simulink model "Dyn_6DoF_v2_0_R2015B"  (R2015b)
settings: Solver=ode4  SolverMode=SingleTasking  StartTime=0.0  StopTime=simInit.TSIM  FixedStep=simInit.dt  MaxStep=simInit.dt  RelTol=1e-3
InitFcn:
  | close all
undefined symbols (not defined in the file): act, base_windspeed, constr, DE2019, DiscIntNeverNeededParam, ENVMT, Lbooth, loiterStates, omega_rate_max, params, simInit, T, winchParameter
libraries: simulink x41, simulink_extras x4, dspsigops x1
(part 6 of 6)

== matlab function Dyn_6DoF_v2_0_R2015B/AirborneSystem/FlightControlSystem/PathFollowingController_SS_3/FlightOnFlatEarth (Retraction&Loitering)/CalculateAttitudeCmds/FlightPathLoopRetraction_Aerodynamic/TrafoPathKin2PathAero ==
  data: Va input; beta input; Vg input; v_w_O input; chi_k input; gamma_k input; chi_a output; gamma_a output
% Copyright 2021 Delft University of Technology
%
% Licensed under the Apache License, Version 2.0 (the "License");
% you may not use this file except in compliance with the License.
% You may obtain a copy of the License at
%
%      http://www.apache.org/licenses/LICENSE-2.0
%
% Unless required by applicable law or agreed to in writing, software
% distributed under the License is distributed on an "AS IS" BASIS,
% WITHOUT WARRANTIES OR CONDITIONS OF ANY KIND, either express or implied.
% See the License for the specific language governing permissions and
% limitations under the License.

function [chi_a, gamma_a] = PathKin2PathAero(Va, beta, Vg, v_w_O, chi_k, gamma_k)
%PathKin2PathAero - transform kinetic path angles into aerodynamic path
%                   angles
%
% Inputs:
%    Va         - Aircraft velocity component on body x axis
%    beta       - Aircraft side slip angle
%    Vg         - Kinetic velocity magnitude
%    v_w_O      - Wind velocity at aircraft in inertial reference frame
%    chi_k      - Kinetic course heading
%    gamma_k    - Kinetic path angle
%
% Outputs:
%    chi_a      - Aerodynamic course heading
%    gamma_a 	- Aerodynamic path angle
%
% Example: [chi_a, gamma_a] = fcn(Va, beta, Vg, v_w_O, chi_k, gamma_k)
%
% Other m-files required: none
% Subfunctions: none
% MAT-files required: none
%
% Author: Sebastian Rapp, Phd.
% Delft University of Technology
% email address: s.rapp@tudelft.nl  

%------------- BEGIN CODE --------------
gamma_a = asin( max( min( (Vg*sin(gamma_k)+v_w_O(3))/(Va+1e-9),1), -1) );
chi_a = beta + chi_k - asin( max( min( 1/(Va*cos(gamma_a)) * (v_w_O(1)*(-sin(chi_k))+v_w_O(2)*cos(chi_k)),1), -1) );
%------------- END CODE --------------
end

== matlab function Dyn_6DoF_v2_0_R2015B/AirborneSystem/ForcesAndTorques/aerodynamic forces FSI/Wing Aero/If Action Subsystem1/FSI/Simple_wing_aero ==
  data: input input double; out output double size=[6,1]; DE2019 parameter; ENVMT parameter
% Copyright 2021 Delft University of Technology
%
% Licensed under the Apache License, Version 2.0 (the "License");
% you may not use this file except in compliance with the License.
% You may obtain a copy of the License at
%
%      http://www.apache.org/licenses/LICENSE-2.0
%
% Unless required by applicable law or agreed to in writing, software
% distributed under the License is distributed on an "AS IS" BASIS,
% WITHOUT WARRANTIES OR CONDITIONS OF ANY KIND, either express or implied.
% See the License for the specific language governing permissions and
% limitations under the License.

function out = simpleAero(input, DE2019, ENVMT)
%simpleAero - Main wing simple aero calculation
%
% Inputs:
%    input  - airspeed, AoA, CL, CD, CM and Croll
%    DE2019 - Aircraft parameters
%    ENVMT  - Environment characteristics
%
% Outputs:
%    out    - 3D forces and moments generated by the wing
%
%
% Author: Sebastian Rapp, Ph.D., Revised by: Dylan Eijkelhof, M.Sc.
% Delft University of Technology
% email address: d.eijkelhof@tudelft.nl
% December 2019; Last revision: 19-March-2021

%-------------	BEGIN CODE	--------------
    V = input(1);
    alpha = input(2);

    q = 0.5*ENVMT.rhos*V^2;

    F_L_main = -input(3)*q*DE2019.S_ref;
    F_D_main = input(4)*q*DE2019.S_ref;
    
    M_y_mw = input(5)*q*DE2019.S_wing*DE2019.c + ...
        (0.25*DE2019.c+DE2019.cog(1))*F_L_main;
    
    c_roll_mw = input(6);
    M_x_mw = (c_roll_mw) * q * DE2019.S_wing * DE2019.b;
    
    F_x_mw = -F_D_main*cos(alpha) - F_L_main*sin(alpha);
    F_z_mw = F_L_main*cos(alpha);


    out = [F_x_mw, 0, F_z_mw, M_x_mw, M_y_mw, 0]';
%-------------	END CODE	--------------
end

== stateflow chart Dyn_6DoF_v2_0_R2015B/AirborneSystem/FlightControlSystem/PathFollowingController_SS_3/FlightOnFlatEarth (Retraction&Loitering)/GuidanceFlatEarth/LoiteringGuidance/Loiter ==
  state initLoiter
    during: [e_track,course_des,valid_transition_region_flag]  = initLoiterGuidance(kp_course_init, p_x_W,p_y_W, pos_OLoiter_W, R_init_loiter, windDir, Vk, validTransReg_start, validTransReg_end);
  (default) -> (junction 217)
  (junction 217) -> initLoiter : [1]
  data: delta function_output; kp_ function_input; p_x_W_ function_input; p_y_W_ function_input; pos_OLoiter_W_ function_input; R_ function_input; windDirection_rad_ function_input; Vk_ function_input; course_des_ function_output; valid_transition_region_flag_ function_output; validTransReg_start_ function_input; validTransReg_end_ function_input; course_des output; p_y_W input; course_k input; p_x_W input; Vk input; kp_course_init parameter; validTransReg_start parameter; validTransReg_end parameter; pos_OLoiter_W parameter; R_init_loiter parameter; valid_transition_region_flag output; e_track output; reset_flag input; windDir input
  function [delta, course_des_,valid_transition_region_flag_]  = initLoiterGuidance(kp_, p_x_W_,p_y_W_, pos_OLoiter_W_, R_, windDirection_rad_, Vk_, validTransReg_start_, validTransReg_end_):
    | % Copyright 2020 Delft University of Technology
    | %
    | % Licensed under the Apache License, Version 2.0 (the "License");
    | % you may not use this file except in compliance with the License.
    | % You may obtain a copy of the License at
    | %
    | %      http://www.apache.org/licenses/LICENSE-2.0
    | %
    | % Unless required by applicable law or agreed to in writing, software
    | % distributed under the License is distributed on an "AS IS" BASIS,
    | % WITHOUT WARRANTIES OR CONDITIONS OF ANY KIND, either express or implied.
    | % See the License for the specific language governing permissions and
    | % limitations under the License. 
    | 
    | function [delta, course_des_,valid_transition_region_flag_]  = initLoiterGuidance(kp_, p_x_W_,p_y_W_, pos_OLoiter_W_, R_, windDirection_rad_, Vk_, validTransReg_start_, validTransReg_end_) 
    | 
    | %#codegen
    | 
    | %% LOITER GUIDANCE: compare with approach where height and ground track is controlled independently
    | p_W_ = [p_x_W_; p_y_W_; 0];
    | 
    | pos_OLoiter_W_(3) = 0;
    | r_circ_W =  pos_OLoiter_W_;
    | 
    | 
    | p_P =  ( p_W_ - r_circ_W );
    | V = [1, 0; 0, 1; 0, 0];
    | p_P = V*((V'*V)\eye(2))*V'*p_P;
    | p_P = p_P / norm(p_P) * R_;
    | 
    | s_star = atan2( p_P(2), p_P(1) );
    | t_P = [-sin(s_star); cos(s_star); 0]*R_;
    | t_W = t_P;% + r_circ_W;
    | t_O = transformFromWtoO(windDirection_rad_, t_W);
    | 
    | p_proj_W =  p_P + r_circ_W;
    | delta_W = p_W_ - p_proj_W;
    | delta = norm( delta_W );
    | 
    | 
    | epx = t_W/norm(t_W);
    | epy = delta_W/norm(delta_W);
    | epz = cross( epx, epy ); epz = epz/norm(epz);
    | 
    | chi_star = atan2(t_O(2), t_O(1));
    | deltaChi = sign(epz(3))*asin( max( min( delta*kp_/Vk_ ,1),-1) );  %atan2( delta, 0.1*R_ );
    | 
    | course_des_ = chi_star + deltaChi;
    | 
    | bearing_O = [cos(course_des_); sin(course_des_); 0];
    | bearing_W = transformFromOtoW(windDirection_rad_, bearing_O);
    | 
    | if s_star > validTransReg_start_ && s_star < validTransReg_end_
    |     valid_transition_region_flag_ = 1;
    | else
    |     valid_transition_region_flag_ = 0;
    | end

== matlab function Dyn_6DoF_v2_0_R2015B/AirborneSystem/6DoFDynamics/MATLAB Function3 ==
  data: v_w_O output; v_w_W input; ENVMT parameter
% Copyright 2021 Delft University of Technology
%
% Licensed under the Apache License, Version 2.0 (the "License");
% you may not use this file except in compliance with the License.
% You may obtain a copy of the License at
%
%      http://www.apache.org/licenses/LICENSE-2.0
%
% Unless required by applicable law or agreed to in writing, software
% distributed under the License is distributed on an "AS IS" BASIS,
% WITHOUT WARRANTIES OR CONDITIONS OF ANY KIND, either express or implied.
% See the License for the specific language governing permissions and
% limitations under the License.

function v_w_O = fcn(v_w_W, ENVMT)

v_w_O = transformFromWtoO(ENVMT.windDirection_rad, v_w_W );
end

== stateflow chart Dyn_6DoF_v2_0_R2015B/GroundSystem_SS_6/StateMachine/checkRetractionCondition ==
  state calcIncrement1
    during: l_tether_predict =l_tether+l_tether-l0;
  state init2
    entry: init_retraction_flag=1;
  state init
    entry: init_retraction_flag=0;
  state calcIncrement
    during: l_tether_predict =l_tether+l_tether-l0;
  state set0length
    entry: l0 = l_tether;
  calcIncrement1 -> (junction 38) : [path_parameter_s >= (3*pi/2-1*pi/180) && path_parameter_s <=3*pi/2+1*pi/180 ]
  init2 -> init : [fm==6]
  (junction 38) -> init2 [order 1] : [l_tether_predict>=l_tether_max*1.15]
  set0length -> calcIncrement1 [order 4] : [path_parameter_s >= (pi/2-1*pi/180) && path_parameter_s <= pi/2+1*pi/180]
  (default) -> init
  set0length -> init [order 2] : [fm==6]
  (junction 38) -> set0length [order 2]
  calcIncrement -> (junction 38) : [path_parameter_s >= (pi/2-1*pi/180) && path_parameter_s <= pi/2+1*pi/180]
  set0length -> init [order 3] : [fm==6]
  init -> set0length : [path_parameter_s >= (pi/2-1*pi/180) && path_parameter_s <= pi/2+1*pi/180 &&fm==5]
  set0length -> calcIncrement [order 1] : [path_parameter_s >= (3*pi/2-1*pi/180) && path_parameter_s <=3*pi/2+1*pi/180 ]
  data: l_tether input; path_parameter_s input; fm input; l0 local; init_retraction_flag output; l_tether_max input; dl local; l_tether_predict local

== matlab function Dyn_6DoF_v2_0_R2015B/AirborneSystem/FlightControlSystem/PathFollowingController_SS_3/FlightOnFlatEarth (Retraction&Loitering)/GuidanceFlatEarth/Retraction_Nav/MATLAB Function1 ==
  data: vel_k_O input; vel_k_h_W output; ENVMT parameter
% Copyright 2021 Delft University of Technology
%
% Licensed under the Apache License, Version 2.0 (the "License");
% you may not use this file except in compliance with the License.
% You may obtain a copy of the License at
%
%      http://www.apache.org/licenses/LICENSE-2.0
%
% Unless required by applicable law or agreed to in writing, software
% distributed under the License is distributed on an "AS IS" BASIS,
% WITHOUT WARRANTIES OR CONDITIONS OF ANY KIND, either express or implied.
% See the License for the specific language governing permissions and
% limitations under the License.

function vel_k_h_W    = fcn(vel_k_O,ENVMT)
%fcn - Calculate horizontal kinetic velocity in wind reference frame
%
% Inputs:
%    vel_k_O    - Kinetic velocity in inertial reference frame
%    ENVMT      - Environment characteristics
%
% Outputs:
%    vel_k_h_W  - Horizontal kinetic velocity magnitude in wind reference frame
%
%
% Author: Sebastian Rapp, Ph.D., Revised by: Dylan Eijkelhof, M.Sc.
% Delft University of Technology
% email address: s.rapp@tudelft.nl
% email address: d.eijkelhof@tudelft.nl
% December 2019; Last revision: 06-October-2020

%-------------	BEGIN CODE	--------------

vel_k_W = transformFromOtoW(ENVMT.windDirection_rad, vel_k_O);

vel_k_h_W = sqrt( vel_k_W(1)^2 + vel_k_W(2)^2 );

%-------------	 END CODE	--------------
end

== matlab function Dyn_6DoF_v2_0_R2015B/AirborneSystem/FlightControlSystem/PathFollowingController_SS_3/FlightOnFlatEarth (Retraction&Loitering)/GuidanceFlatEarth/Retraction_Nav/circle_vertical ==
  data: pos_O input; arcsize input; Vk_desired output; V_ro input; l_actual input; d_gt output; d output; chi_k_cmd output; flag_pos_y_W output; switch_WP_x_W output; gamma_k_cmd output; pos_init_retraction_O input; transition_flag output; ENVMT parameter; v_k_tot input; constr parameter; params parameter; vk_xy input; arcP_old input; transition_flag_old input; arcP output
% Copyright 2021 Delft University of Technology
%
% Licensed under the Apache License, Version 2.0 (the "License");
% you may not use this file except in compliance with the License.
% You may obtain a copy of the License at
%
%      http://www.apache.org/licenses/LICENSE-2.0
%
% Unless required by applicable law or agreed to in writing, software
% distributed under the License is distributed on an "AS IS" BASIS,
% WITHOUT WARRANTIES OR CONDITIONS OF ANY KIND, either express or implied.
% See the License for the specific language governing permissions and
% limitations under the License.

function [Vk_desired,d_gt, d, chi_k_cmd,flag_pos_y_W,switch_WP_x_W, gamma_k_cmd, transition_flag,arcP] = ...
    slope_vert_arc(pos_O, arcsize, V_ro, l_actual, pos_init_retraction_O, ENVMT, v_k_tot, constr, params, ...
    vk_xy, arcP_old, transition_flag_old)
%slope_navigator - Navigation on slope during retraction
%
% Inputs:
%    pos_O                  - Aircraft position in inertial reference frame
%    arcsize                - Matrix to pre-allocate retraction path params
%    V_ro                   - Tether reel-out speed
%    l_actual               - Actual tether length
%    pos_init_retraction_O  - Aircraft position at start of retraction in
%                             inertial reference frame
%    ENVMT                  - Environment characteristics
%    v_k_tot                - Magnitude of kinetic velocity
%    constr                 - Constraint, minimum altitude
%    params                 - Controller parameters and Fig8 shape
%    vk_xy                  - Horizontal kinetic velocity magnitude in wind
%                             reference frame
%    arcP_old               - Retraction shape calculated at first
%                             retraction time step
%    transition_flag_old    - Old transition from retraction to traction flag
%
% Outputs:
%    Vk_desired      - Desired kinetic velocity to have a straight tether
%                      at target
%    d_gt            - Distance to ground track
%    d               - Distance to slope
%    chi_k_cmd       - Desired Course angle
%    flag_pos_y_W    - Flag to determine on which side it needs to go into
%                      traction
%    switch_WP_x_W   - X coordinate of the retraction target to transition
%    gamma_k_cmd     - Desired path angle
%    transition_flag - Transition from retraction to traction flag
%    arcP            - Retraction path discretisation points
%
% Other m-files required: none
% Subfunctions: calc_retARCi - Determine arc shape
% MAT-files required: none
%
% Author: Sebastian Rapp, Ph.D., Revised by: Dylan Eijkelhof, M.Sc.
% Delft University of Technology
% email address: s.rapp@tudelft.nl
% email address: d.eijkelhof@tudelft.nl
% December 2019; Last revision: 19-March-2021

%-------------	BEGIN CODE	--------------

pos_init_retraction_W = transformFromOtoW(ENVMT.windDirection_rad, pos_init_retraction_O);
pos_W = transformFromOtoW(ENVMT.windDirection_rad, pos_O);

if pos_init_retraction_W(2) > 0 
    flag_pos_y_W = 1;%1
else
    flag_pos_y_W = 0;%0
end

%% outer point lemniscate
Lbooth.b = params.b_booth;
Lbooth.a = params.b_booth*params.a_booth;
Lbooth.phi0 = params.transition_phi*pi/180;
l_tether_min = params.l_tether_min*params.l_tether_max;
[Lem] = updateBoothLemniscate(l_tether_min,Lbooth);
if flag_pos_y_W
    s = pi/2;
else
    s = 3/2*pi; 
end
long_P = Lem.b * sin(s) ./( 1+(Lem.a/Lem.b*cos(s)).^2 );
lat_P = Lem.a * sin(s).*cos(s) ./ ( 1+(Lem.a/Lem.b*cos(s)).^2 );
p_P = [ cos(long_P).*cos(lat_P);sin(long_P).*cos(lat_P);sin(lat_P)]*l_tether_min;
M_WP = [cos(Lbooth.phi0),0, -sin(Lbooth.phi0);0, 1, 0;  sin(Lbooth.phi0),0, cos(Lbooth.phi0)];  
p_W = M_WP * p_P; 
%%

p_W(1) = -params.x_arcEnd;
p_W(2) = p_W(2)*1.3;

target_W = p_W;% params.target_retraction_W;
switch_WP_x_W = p_W(1);
switch_WP_y_W = p_W(2);


switch_WP_W = [switch_WP_x_W;switch_WP_y_W;0];

% min tether length before the turn
if l_tether_min^2 - switch_WP_x_W^2 - switch_WP_y_W^2 > 0
    z_transition = max( sqrt( l_tether_min^2 - switch_WP_x_W^2 - switch_WP_y_W^2 ), constr.min_altitude_pc); % min. attitude has higher priority then min. tether length
else
    z_transition = constr.min_altitude_pc;
end

Pstart = pos_init_retraction_W;
Ptarget = [target_W(1),target_W(2), z_transition]';
euc_dist = norm(Pstart-Ptarget);
R = params.arc1*(euc_dist/2+1); %Arbitrary value of arc radius, bigger --> slope
if all(arcP_old==arcsize)
    %only calculate at start of retraction
    [arcP] = calc_retARCi(Pstart,Ptarget,params.arc1,'v','up',arcsize);
else
    arcP = arcP_old;
end
dist = sqrt((arcP(3,:) - pos_W(3)).^2 + (arcP(2,:) - pos_W(2)).^2 + (arcP(1,:) - pos_W(1)).^2);
[~,idx] = min(dist,[],2); % index for the closest points, i.e. those with min distance.

if idx == size(arcP,2)
    groundtrack_bearing_W = arcP(:,size(arcP,2)) - arcP(:,size(arcP,2)-1);
else
    groundtrack_bearing_W = arcP(:,idx+1) - arcP(:,idx);
end

if pos_W(1) <= p_W(1) || transition_flag_old
    transition_flag = 1;
    groundtrack_bearing_W = arcP(:,size(arcP,2)) - arcP(:,size(arcP,2)-1);
    groundtrack_bearing_O = transformFromWtoO(ENVMT.windDirection_rad, groundtrack_bearing_W);
    chi_k_cmd = atan2( groundtrack_bearing_O(2), groundtrack_bearing_O(1) );
    groundtrack_bearing_W(3) = 0;
    
    % relative position
    pos_rel_gt_W = pos_W - pos_init_retraction_W;
    pos_rel_gt_W(3) = 0;
    
    % projection onto groundtrack
    p_proj_W = pos_rel_gt_W'*groundtrack_bearing_W / norm( groundtrack_bearing_W )^2 * groundtrack_bearing_W;
    % distance 2 ground track
    d_gt = norm( pos_rel_gt_W - p_proj_W );

else
    transition_flag = 0;
    groundtrack_bearing_O = transformFromWtoO(ENVMT.windDirection_rad, groundtrack_bearing_W);
    chi_k_cmd = atan2( groundtrack_bearing_O(2), groundtrack_bearing_O(1) );
    
    % Desired ground track
    groundtrack_bearing_W = arcP(:,idx) - pos_init_retraction_W;
    groundtrack_bearing_W(3) = 0;
    
    % relative position
    pos_rel_gt_W = pos_W - pos_init_retraction_W;
    pos_rel_gt_W(3) = 0;
    
    % projection onto groundtrack
    p_proj_W = pos_rel_gt_W'*groundtrack_bearing_W / norm( groundtrack_bearing_W )^2 * groundtrack_bearing_W;
    % distance 2 ground track
    d_gt = norm( pos_rel_gt_W - p_proj_W );
    z = cross( groundtrack_bearing_W,pos_rel_gt_W );
    
    delta_chi = sign(z(3)) * asin( max( min( params.kp_delta_course*d_gt / vk_xy, 1),-1) );
    
    chi_k_cmd = chi_k_cmd + delta_chi;
end

%% arc length of transition circle until transition point 

dh = pos_init_retraction_W(3) - z_transition;
ds = sqrt( ( switch_WP_x_W - pos_init_retraction_W(1))^2 +  ( switch_WP_y_W - pos_init_retraction_W(2))^2 ); 
gamma_k_star =  atan2( -dh,ds );

gs_direction_W = [switch_WP_W(1) - pos_init_retraction_W(1);switch_WP_W(2) - pos_init_retraction_W(2);-dh];

% Current relative position vector
p_rel_W = pos_W - pos_init_retraction_W;

% projection onto retraction slope
p_proj_W = p_rel_W'*gs_direction_W / norm( gs_direction_W )^2 * gs_direction_W;

% distance to slope
d = norm( p_rel_W - p_proj_W );

if transition_flag
    d = abs( pos_W(3) - z_transition );
    gamma_k_cmd = 0;
else 
    % check if above or below glide slope
    z = cross( gs_direction_W,p_rel_W );
    sign_deltaGamma = sign(z(2));
    gamma_k_cmd = gamma_k_star - asin( max( min(params.kp_delta_gamma*d*sign_deltaGamma/(v_k_tot+1e-3), pi/6), -pi/6) );
end


l_desired = norm([target_W(1),target_W(2), z_transition]);
if V_ro>0
    t_retract = (l_actual - l_desired)/(25);
else
    t_retract = (l_actual - l_desired)/(-V_ro);
end
ang1 = 2* asin(((norm(pos_W-[target_W(1),target_W(2), z_transition]'))/2)/R);
arc_dist = R*ang1;
Vk_desired = arc_dist/t_retract;
%-------------	 END CODE	--------------
end

function [arcP] = calc_retARCi(Pstartf,Ptargetf,Rmultiplier,direction,updown,arcsize)

euc_dist = norm(Pstartf-Ptargetf);
R = Rmultiplier*(euc_dist/2+1); %Arbitrary value of arc radius, bigger --> tighter curve
u = (Pstartf-Ptargetf)/norm(Pstartf-Ptargetf); % unit vector in direction of slope
Pm = (Pstartf+Ptargetf)/2;

if Pstartf(2)>0
    v = [-u(2)/u(1);1;0];
else
    v = [u(2)/u(1);-1;0];
end
v = v/norm(v);
n = cross(v,u);
    
W_u = [0,-u(3),u(2);u(3), 0, -u(1);-u(2),u(1),0];
Rotu_180 = eye(3)+2*W_u^2;

if strcmp(updown,'up')
    if n(3) < 0
        n = Rotu_180*n;
    end
elseif strcmp(updown,'down')
    if n(3) > 0
        n = Rotu_180*n;
    end
end

if strcmp(direction,'v')
    v_temp = n;
    n = v;
    v = v_temp;
end

W = [0,-n(3),n(2);n(3), 0, -n(1);-n(2),n(1),0];
h = R-sqrt(R^2-(euc_dist/2)^2);
Center = Pm + (h-R)*v;
ang = 2* asin((euc_dist/2)/R);

tlist=linspace(0,1,size(arcsize,2));
arcP = zeros(3,numel(tlist));
for i = 1:numel(tlist)
    Rotn = eye(3)+sin(-ang/2+tlist(i)*ang)*W+(2*sin((-ang/2+tlist(i)*ang)/2)^2)*W^2;
    arcP(:,i) = Center + Rotn*v*R;
end

if norm(Pstartf-arcP(:,1))>1
    arcP = fliplr(arcP);
end

end

== matlab function Dyn_6DoF_v2_0_R2015B/AirborneSystem/FlightControlSystem/PathFollowingController_SS_3/FlightOnSphere (Traction)/FlightPathLoopTraction/EstimatePlantResponse/MATLAB Function ==
  data: F_t input; dphi input; mu_k input; chi_dot_real output; gamma_dot_real output; DE2019 parameter; chi_k input; gamma_k input; pos_O input; v_k_B input; airdata input; ENVMT parameter
% Copyright 2021 Delft University of Technology
%
% Licensed under the Apache License, Version 2.0 (the "License");
% you may not use this file except in compliance with the License.
% You may obtain a copy of the License at
%
%      http://www.apache.org/licenses/LICENSE-2.0
%
% Unless required by applicable law or agreed to in writing, software
% distributed under the License is distributed on an "AS IS" BASIS,
% WITHOUT WARRANTIES OR CONDITIONS OF ANY KIND, either express or implied.
% See the License for the specific language governing permissions and
% limitations under the License.

function [chi_dot_real, gamma_dot_real] = est_pathangles(F_t, dphi, mu_k,DE2019,chi_k,gamma_k, pos_O, v_k_B, airdata,ENVMT)
%est_pathangles - Estimate plant response
%
% Inputs:
%    F_t     - Tether set point
%    dphi    - Set to 0, not used currently
%    mu_k    - Roll angle
%    DE2019  - Aircraft characteristics
%    chi_k   - Course angle
%    gamma_k - Path angle
%    pos_O   - Aircraft position in inertial reference frame
%    v_k_B   - Kinetic velocity in body reference frame
%    airdata - Airspeed, aoa, sideslip
%    ENVMT   - Enivronment characteristics
%
% Outputs:
%    chi_dot_real    - Course angle rate of change
%    gamma_dot_real  - Path angle rate of change
%
%
% Author: Sebastian Rapp, Ph.D., Revised by: Dylan Eijkelhof, M.Sc.
% Delft University of Technology
% email address: s.rapp@tudelft.nl
% email address: d.eijkelhof@tudelft.nl
% December 2019; Last revision: 06-October-2020

%-------------	BEGIN CODE	--------------

Va = airdata(1); 
alpha = airdata(2); 
vk = norm(v_k_B); 
CL = DE2019.CL0 + DE2019.CL_alpha*alpha; 

Lrq = 0.5 * Va^2 * 1.225 * DE2019.S_wing * CL; 

c_chi_k = cos(chi_k); 
c_gamma_k = cos(gamma_k); 
s_chi_k = sin(chi_k); 
s_gamma_k = sin(gamma_k); 


M_KO = [ c_chi_k*c_gamma_k, s_chi_k*c_gamma_k, -s_gamma_k; 
    -s_chi_k, c_chi_k, 0; 
    c_chi_k*s_gamma_k, s_chi_k*s_gamma_k, c_gamma_k];

F_g_t_K = M_KO * ( [0;0;DE2019.mass*ENVMT.g] -F_t*pos_O/norm(pos_O) );

f_bar_z_K = -Lrq/sqrt(1+(tan(mu_k-dphi))^2); 

f_bar_y_K = -f_bar_z_K * tan( mu_k - dphi );

chi_dot_real = 1/cos(gamma_k)/vk/DE2019.mass  * ( f_bar_y_K + F_g_t_K(2) );
gamma_dot_real = -1/vk/DE2019.mass * ( f_bar_z_K + F_g_t_K(3) );

%-------------	 END CODE	--------------
end

== matlab function Dyn_6DoF_v2_0_R2015B/AirborneSystem/FlightControlSystem/PathFollowingController_SS_3/FlightOnSphere (Traction)/FlightPathLoopTraction/MATLAB Function ==
  data: L_rq output; airdata input; DE2019 parameter; constr parameter; ENVMT parameter
% Copyright 2021 Delft University of Technology
%
% Licensed under the Apache License, Version 2.0 (the "License");
% you may not use this file except in compliance with the License.
% You may obtain a copy of the License at
%
%      http://www.apache.org/licenses/LICENSE-2.0
%
% Unless required by applicable law or agreed to in writing, software
% distributed under the License is distributed on an "AS IS" BASIS,
% WITHOUT WARRANTIES OR CONDITIONS OF ANY KIND, either express or implied.
% See the License for the specific language governing permissions and
% limitations under the License.

function L_rq = fcn(airdata, DE2019, constr, ENVMT)
%fcn - Calculate required lift force
%
% Inputs:
%    airdata     - Airspeed, aoa, sideslip angle
%    DE2019     - Aircraft characteristics
%    constr     - Constraint, maximum lift
%
% Outputs:
%    L_rq    - Required lift
%
% Author: Sebastian Rapp, Ph.D., Revised by: Dylan Eijkelhof, M.Sc.
% Delft University of Technology
% email address: s.rapp@tudelft.nl
% email address: d.eijkelhof@tudelft.nl
% December 2019; Last revision: 06-October-2020

%-------------	BEGIN CODE	--------------
L_rq =  min( 0.5*ENVMT.rhos*DE2019.S_wing*airdata(1)^2 * (DE2019.CL0+DE2019.CL_alpha*airdata(2) ),constr.F_T_max); % max. negative lift
%-------------	 END CODE	--------------
end

== matlab function Dyn_6DoF_v2_0_R2015B/AirborneSystem/FlightControlSystem/PathFollowingController_SS_3/FlightOnSphere (Traction)/FlightPathLoopTraction/inversionPathDynamics ==
  data: Ft_set input; nu_chi_k input; mu_a output; nu_gamma_k input; F_a_B_est input; DE2019 parameter; pos_O input; chi_k input; gamma_k input; v_k_B input; airdata input; constr parameter; mu_k_c output; alpha_rq output; dphi output; L_rq output; L_rq_old input; mu_a_old input; ENVMT parameter
% Copyright 2021 Delft University of Technology
%
% Licensed under the Apache License, Version 2.0 (the "License");
% you may not use this file except in compliance with the License.
% You may obtain a copy of the License at
%
%      http://www.apache.org/licenses/LICENSE-2.0
%
% Unless required by applicable law or agreed to in writing, software
% distributed under the License is distributed on an "AS IS" BASIS,
% WITHOUT WARRANTIES OR CONDITIONS OF ANY KIND, either express or implied.
% See the License for the specific language governing permissions and
% limitations under the License.

function [mu_a,mu_k_c,alpha_rq,dphi,L_rq] = InversePathDynamics(  Ft_set, nu_chi_k, nu_gamma_k, F_a_B_est,DE2019,pos_O,...
     chi_k, gamma_k, v_k_B, airdata, constr, L_rq_old, mu_a_old,ENVMT)
%InversePathDynamics - Calculated desired roll and pitch angles 
%
% Inputs:
%    Ft_set     - Tether force set point
%    nu_chi_k   - Course angle error
%    nu_gamma_k - Path angle error
%    F_a_B_est  - Aerodynamic forces in body reference frame
%    DE2019     - Aircraft characteristics
%    pos_O      - Aircraft position in inertial reference frame
%    chi_k      - Course angle
%    gamma_k    - Path angle
%    v_k_B      - Kinetic velocity
%    airdata    - Airspeed, aoa and sideslip angle
%    constr     - Dynamic constraints
%    L_rq_old   - Old required lift
%    mu_a_old   - Old roll angle
%    ENVMT      - Environment characteristics
%
% Outputs:
%    mu_a     - Desired aerodynamic roll angle
%    mu_k_c   - Kinetic roll angle
%    alpha_rq - Desired pitch angle
%    dphi     - Currently set to 0, not used anymore
%    L_rq     - Required lift
%
% Author: Sebastian Rapp, Ph.D., Revised by: Dylan Eijkelhof, M.Sc.
% Delft University of Technology
% email address: s.rapp@tudelft.nl
% email address: d.eijkelhof@tudelft.nl
% December 2019; Last revision: 06-October-2020

%-------------	BEGIN CODE	--------------
%% Initialise parameters for codegen
mu_a = 0;
mu_k_c = 0;
alpha_rq = 0;
dphi = 0;
v_k = 0;
L_rq = 0;
fbar_z_K = 0;
fbar_z_K_is = 0;

%%
f_t = Ft_set; 
mu_k_max = constr.mu_k_max;

beta_a = airdata(3); 

alpha_k = asin( v_k_B(3)/norm(v_k_B) ); 
beta_k = atan2( v_k_B(2), v_k_B(1) ); 

v_k = norm(v_k_B); 

c_chi_k = cos(chi_k); 
c_gamma_k = cos(gamma_k); 
s_chi_k = sin(chi_k); 
s_gamma_k = sin(gamma_k); 


M_KO = [ c_chi_k*c_gamma_k, s_chi_k*c_gamma_k, -s_gamma_k; 
    -s_chi_k, c_chi_k, 0; 
    c_chi_k*s_gamma_k, s_chi_k*s_gamma_k, c_gamma_k];

f_a_x_B = F_a_B_est(1); 
f_a_y_B = F_a_B_est(2); 
f_a_z_B = F_a_B_est(3); 


f_a_y_Kbar = -cos(alpha_k)*sin(beta_k)*f_a_x_B + cos(beta_k)*f_a_y_B - sin(alpha_k)*sin(beta_k)*f_a_z_B; 
f_a_z_Kbar = -sin(alpha_k)*f_a_x_B + cos(alpha_k)*f_a_z_B; 

f_t_K = -M_KO * pos_O/norm(pos_O)*f_t; 

fbar_y_K = DE2019.mass*nu_chi_k*cos(gamma_k)*v_k - f_t_K(2); 
fbar_z_K = -DE2019.mass*nu_gamma_k*v_k - cos(gamma_k)*DE2019.mass*ENVMT.g - f_t_K(3);

dphi = 0 * atan( f_a_y_Kbar / f_a_z_Kbar ); % this might be important at high wind speeds

mu_k_c = atan2( fbar_y_K, -fbar_z_K ) + dphi; 
fbar_y_K =  -fbar_z_K * tan( mu_k_c - dphi );

L_rq = min( sqrt( fbar_y_K^2 + fbar_z_K^2 )); % constraint by max. tether force e.g. structural limit

% limit mu_k: We do this for now directly: if we assume that the kite is in
% the tangential plane this corresponds well to the limits for phi_tau

mu_k_c = max( min( mu_k_c, mu_k_max), -mu_k_max); 

mu_a = mu_k_c;

% hold old bank angle if required lift is very small, avoid agressive
% banking for small absolute values of L i.e. for small values inaccuracies
% like numerical inaccuracies have a large impact on the mu_a_c.
if abs(L_rq) <= 100
    mu_a = mu_a_old;
end

% for large bank angle changes only adapt the lift if close to the current
% lift. The longitudional dynamic is faster, hence if we command large bank
% angles this would result in a large lift which would first create a large
% curvature in the longi plane before the actual curvature in the lateral
% plan is achieved.
if abs( mu_a - mu_a_old ) > constr.max_delta_mu
    L_rq = L_rq_old;
end

CL_rq = 2*L_rq / ( ENVMT.rhos*DE2019.S_wing*airdata(1)^2 );
alpha_rq = (CL_rq - DE2019.CL0)/DE2019.CL_alpha; 

%-------------	 END CODE	--------------
end

== matlab function Dyn_6DoF_v2_0_R2015B/AirborneSystem/FlightControlSystem/PathFollowingController_SS_3/FlightOnSphere (Traction)/Navigator/LissajousFigure8Following ==
  data: chi_k_ideal output; gamma_k_ideal output; chi_dot output; gamma_dot output; delta_ct output; pathAngles input; pos_W input; v_w_vec input; v_O_vec input; ENVMT parameter; long input; lat input; Lbooth parameter; params parameter; gamma_tau_dot input; gamma_tau_cmd input; PHI_BOOTH input; sub_flight_state input; sol output; sol_old input
% Copyright 2021 Delft University of Technology
%
% Licensed under the Apache License, Version 2.0 (the "License");
% you may not use this file except in compliance with the License.
% You may obtain a copy of the License at
%
%      http://www.apache.org/licenses/LICENSE-2.0
%
% Unless required by applicable law or agreed to in writing, software
% distributed under the License is distributed on an "AS IS" BASIS,
% WITHOUT WARRANTIES OR CONDITIONS OF ANY KIND, either express or implied.
% See the License for the specific language governing permissions and
% limitations under the License.

function [chi_k_ideal, gamma_k_ideal, chi_dot, ...
    gamma_dot, delta_ct, sol] = fig8_navigator(pathAngles, ...
    pos_W,v_w_vec, v_O_vec, ENVMT, long, lat,Lbooth,params,gamma_tau_dot, ...
    gamma_tau_cmd,PHI_BOOTH, sub_flight_state, sol_old)
%fig8_navigator - Unlinke the other modules this module directly calculates
%                 the desired course and path angle rate
%
% Inputs:
%    pathAngles     - Course and path angles
%    pos_W          - Aircraft position in wind reference frame
%    v_w_vec        - Wind speed in wind reference frame
%    v_O_vec        - Kinetic velocity in inertial reference frame
%    ENVMT          - Environment characteristics
%    long           - Logtitude (ground station in sphere centre)
%    lat            - Latitude (ground station in sphere centre)
%    Lbooth         - Structure initialisation, parameters not used
%    params         - Controller parameters and Fig8 shape
%    gamma_tau_dot  - Input 0!
%    gamma_tau_cmd  - Input 0!
%    PHI_BOOTH      - Elevation angle
%    sol_old        - Old point on fig8 (0->2pi)
%
% Outputs:
%    chi_k_ideal     - Desired kinetic course angle
%    gamma_k_ideal   - Desired kinetic path angle
%    chi_dot         - Course angle rate of change
%    gamma_dot       - Path angle rate of change
%    delta_ct        - Cross-track error
%    sol             - Point on fig8 (0->2pi)
%
% Author: Sebastian Rapp, Ph.D., Revised by: Dylan Eijkelhof, M.Sc.
% Delft University of Technology
% email address: s.rapp@tudelft.nl
% email address: d.eijkelhof@tudelft.nl
% December 2019; Last revision: 06-October-2020

%-------------	BEGIN CODE	--------------

windDirection_rad = ENVMT.windDirection_rad;

b_booth = params.b_booth;
a_booth = params.a_booth;

% total kinematic velocity
Vtot = sqrt( v_O_vec'*v_O_vec );

% transform position from NEDframe (O) into Windframe (W)
phi_p_mean = PHI_BOOTH;  
M_WP = [cos(phi_p_mean),0, -sin(phi_p_mean);0, 1, 0; sin(phi_p_mean),0, cos(phi_p_mean)];
pos_P = M_WP' * pos_W; 

distanceOrigin = norm(pos_P);

% Booth Lemniscate
Lbooth.a = a_booth*b_booth; % height
Lbooth.b = b_booth; % length
Lbooth.phi0 = PHI_BOOTH; %phi0_booth*pi/180;

[Lem] = updateBoothLemniscate(distanceOrigin,Lbooth);
direction = -1;

[ sol,p_C_P] = getTargetOnBoothNewton2(Lem, pos_P, sol_old, distanceOrigin, direction);
[t_P,DtDs_P,~,~,~] = getBoothInfos2(sol,Lem, direction);
t = M_WP * t_P; 
DtDs = M_WP * DtDs_P; 
p_C_W = M_WP * p_C_P; 

% ---- I Think everything below is curve independent -----

% Step 2: Calculate distance to closest point
delta = acos( min( max( pos_W'/norm(pos_W) * p_C_W/norm(p_C_W), -1),1 ) );
delta_ct = delta * distanceOrigin;

% Step 3: Calculate the perpendicular course
[ ~, delta_vec, ~] = calcCourse2ClosestPoint( p_C_W, pos_W );
% delta_ct_signed = bearing_sign*delta;

% Step 3.5: Parallel transport of vectors at the path point to the kite
% position
t_rot = doRodriguesRotation(pos_W, p_C_W, t);
t_rot_T = transformFromWtoTau(long, lat, t_rot);
chi_parallel = atan2( t_rot_T(2), t_rot_T(1) );

chi = atan2( v_O_vec(2), v_O_vec(1) ); 
gamma = -asin( v_O_vec(3)/norm(v_O_vec) ); 
bearing_is_O = [cos(chi)*cos(gamma);
    sin(chi)*cos(gamma);
    -sin(gamma)];
bearing_is_tau = transformFromWtoTau( long, lat, transformFromOtoW(windDirection_rad, bearing_is_O));
chi_tau_is = atan2( bearing_is_tau(2), bearing_is_tau(1));
gamma_tau_is = -asin( bearing_is_tau(3) / norm( bearing_is_tau ) );

% Step 4: Calculate commanded course in tangential plane
% and determine the ideal bearing vector
V_k_tau = [cos(chi_tau_is)*cos(gamma_tau_is),sin(chi_tau_is)*cos(gamma_tau_is),0]*Vtot/distanceOrigin; 
delta0 = min(params.delta0_slope*norm(V_k_tau),0.1)+params.delta0_offset;%0.0025*max( min( norm(V_k_tau), 35),25) ;

[chi_tau, ~,~, Delta_chi_dot, ~] = calculateCommandedCourse2(t_rot,delta_vec, delta, delta0, chi_parallel, p_C_W, pos_W,v_w_vec, chi_tau_is);

% Step 5: Predict the required course rate due to the path curvature
[chi_tau_dot_predict] = predictChiDotRequ(long,lat,v_w_vec, pos_W,p_C_W, t, DtDs,chi_parallel );

gamma_tau = gamma_tau_cmd;

v_tau = [cos(chi_tau)*cos(gamma_tau); 
         sin(chi_tau)*cos(gamma_tau); 
        -sin(gamma_tau)]*Vtot;

v_w_vec_ideal = transformFromTautoW(long,lat, v_tau);
bearing_O = transformFromWtoO(windDirection_rad, v_w_vec_ideal); 
% if sub_flight_state== 5
%     chi_k_ideal = 0;
%     gamma_k_ideal = 0;
% else
chi_k_ideal = atan2( bearing_O(2), bearing_O(1) );
gamma_k_ideal = -asin( bearing_O(3)/norm(bearing_O) );
% end

% Step 6: Calculate the required course rate in the tangential plane 
nu_ref = chi_tau_dot_predict + Delta_chi_dot;

%%
chi = pathAngles(1); 
gamma = pathAngles(2);
chi_tau_dot_cmd = nu_ref ;
% 
% if sub_flight_state== 5
%     chi_dot = 0;
%     gamma_dot = 0;
% else
[chi_dot, gamma_dot] = getChiDotGammaDotOK(ENVMT.windDirection_rad,lat,long, v_w_vec,...
    chi_tau_dot_cmd, norm(pos_W),chi, gamma, v_w_vec_ideal, pos_W,gamma_tau,gamma_tau_dot);
% end
%-------------	 END CODE	--------------
end

== matlab function Dyn_6DoF_v2_0_R2015B/AirborneSystem/FlightControlSystem/PathFollowingController_SS_3/FlightOnSphere (Traction)/Navigator/calcualteCourseErrorAndWrap1 ==
  data: chi_ref input; e_course output; chi input
% Copyright 2021 Delft University of Technology
%
% Licensed under the Apache License, Version 2.0 (the "License");
% you may not use this file except in compliance with the License.
% You may obtain a copy of the License at
%
%      http://www.apache.org/licenses/LICENSE-2.0
%
% Unless required by applicable law or agreed to in writing, software
% distributed under the License is distributed on an "AS IS" BASIS,
% WITHOUT WARRANTIES OR CONDITIONS OF ANY KIND, either express or implied.
% See the License for the specific language governing permissions and
% limitations under the License.

function e_course = course_error(chi_ref, chi)
%course_error - Calculate the error between commanded and actual course angle
%
% Inputs:
%    chi_ref  - Required chi
%    chi      - Actual chi
%
% Outputs:
%    e_course - Course (heading) error
%
% Example: 
%    
%
% Author: Sebastian Rapp, Ph.D., Revised by: Dylan Eijkelhof, M.Sc.
% Delft University of Technology
% email address: s.rapp@tudelft.nl
% email address: d.eijkelhof@tudelft.nl
% December 2019; Last revision: 06-October-2020

%-------------	BEGIN CODE	--------------
%#codegen
% The vectors are lying in the tangential plane attached to the current
% position on the small earth.
p_bearing_vec   = [cos(chi); sin(chi); 0];
p_bearing_vec   = p_bearing_vec/norm(p_bearing_vec); 

ref_bearing_vec = [cos(chi_ref); sin(chi_ref); 0];
ref_bearing_vec = ref_bearing_vec/norm(ref_bearing_vec); 

e_z = cross( ref_bearing_vec, p_bearing_vec ); 

dot_product = dot( ref_bearing_vec, p_bearing_vec ); 
if dot_product > 1 
	dot_product = 1; 
end
if dot_product < -1 
	dot_product = -1; 
end

e_course = - sign( e_z(3) ) * acos( max(min(dot_product,1),-1) );
%-------------	 END CODE	--------------
end

== stateflow chart Dyn_6DoF_v2_0_R2015B/AirborneSystem/FlightControlSystem/PathFollowingController_SS_3/FlightOnSphere (Traction)/Select_init_sol_for_pathfollowing ==
  state Pumping
    entry: sol_init = pi/2;
    %entry: sol_init = 45/180*pi;
  state Init
    entry: sol_init = x;
  state Pumping1
    entry: sol_init = 3*pi/2;
    %entry: sol_init = 225/180*pi;
  (junction 20) -> (junction 21)
  Pumping -> (junction 20) : [fm == 5]
  (junction 21) -> Init
  (default) -> Init
  (junction 17) -> Pumping [order 1] : [flag_pos_y_W==1]
  Init -> (junction 17) : [fm == 6 ]
  (junction 17) -> (junction 12) [order 2] : [flag_pos_y_W==0]
  (junction 24) -> Init
  (junction 12) -> Pumping1
  Pumping1 -> (junction 25) : [fm == 5]
  (junction 25) -> (junction 24)
  data: x input; fm input; sol_init output; flag_pos_y_W input

== matlab function Dyn_6DoF_v2_0_R2015B/AirborneSystem/ForcesAndTorques/aerodynamic forces FSI/Elevator Aero/Elevator_aero ==
  data: input input double; out output double size=[6,1]; DE2019 parameter; ENVMT parameter
% Copyright 2021 Delft University of Technology
%
% Licensed under the Apache License, Version 2.0 (the "License");
% you may not use this file except in compliance with the License.
% You may obtain a copy of the License at
%
%      http://www.apache.org/licenses/LICENSE-2.0
%
% Unless required by applicable law or agreed to in writing, software
% distributed under the License is distributed on an "AS IS" BASIS,
% WITHOUT WARRANTIES OR CONDITIONS OF ANY KIND, either express or implied.
% See the License for the specific language governing permissions and
% limitations under the License.

function out = simpleAero(input, DE2019, ENVMT)
%simpleAero - Elevator simple aero calculation
%
% Inputs:
%    input  - airspeed, AoA, sideslip, CL and CD
%    DE2019 - Aircraft parameters
%    ENVMT  - Environment characteristics
%
% Outputs:
%    out    - 3D forces and moments generated by the elevator
%
%
% Author: Sebastian Rapp, Ph.D., Revised by: Dylan Eijkelhof, M.Sc.
% Delft University of Technology
% email address: d.eijkelhof@tudelft.nl
% December 2019; Last revision: 19-March-2021

%-------------	BEGIN CODE	--------------
    V = input(1);
    alpha = input(2);
    beta = input(3);

    q = 0.5*ENVMT.rhos*V^2;

    F_L_el = -input(4)*q*DE2019.S_el;
    F_D_el = -input(5)*q*DE2019.S_el;

    F_x_s = F_D_el*cos(alpha)*cos(beta) - F_L_el*sin(alpha)*cos(beta);
    F_y_s = 0;
    F_z_s = F_L_el*cos(alpha);

    M_x_s = 0;
    M_y_s = F_L_el*(DE2019.x_el+DE2019.c_el*0.25);
    M_z_s = 0;

    out = [F_x_s, F_y_s, F_z_s, M_x_s, M_y_s, M_z_s]';
%-------------	END CODE	--------------
end

== matlab function Dyn_6DoF_v2_0_R2015B/AirborneSystem/FlightControlSystem/AttitudeAndRateLoop/RateLoop/Rate_Loop/Hedging/InversionRotationalDynamics1 ==
  data: nu_p_hat output; Moments input; p input; q input; r input; DE2019 parameter; nu_q_hat output; nu_r_hat output
% Copyright 2021 Delft University of Technology
%
% Licensed under the Apache License, Version 2.0 (the "License");
% you may not use this file except in compliance with the License.
% You may obtain a copy of the License at
%
%      http://www.apache.org/licenses/LICENSE-2.0
%
% Unless required by applicable law or agreed to in writing, software
% distributed under the License is distributed on an "AS IS" BASIS,
% WITHOUT WARRANTIES OR CONDITIONS OF ANY KIND, either express or implied.
% See the License for the specific language governing permissions and
% limitations under the License.

function [nu_p_hat, nu_q_hat, nu_r_hat] = hedging_rot_inv(Moments, p, q, r, DE2019)
%hedging_rot_inv - Expected error after inversion
%
% Inputs:
%    Moments   - Roll, pitch and yaw moment
%    p         - Roll rate
%    q         - Pitch rate
%    r         - Yaw rate
%    DE2019    - Aircraft parameters
%
% Outputs:
%    nu_p_hat  - Expected roll rate error
%    nu_q_hat  - Expected pitch rate error
%    nu_r_hat  - Expected yaw rate error
%
% Other m-files required:   none
% Subfunctions:             none
% MAT-files required:       none
%
% Author: Sebastian Rapp, Ph.D., Revised by: Dylan Eijkelhof, M.Sc.
% Delft University of Technology
% email address: d.eijkelhof@tudelft.nl
% December 2019; Last revision: 19-March-2021

%------------- BEGIN CODE --------------
 
L = Moments(1); 
M = Moments(2); 
N = Moments(3); 

Jx =  DE2019.J(1,1); 
Jy =  DE2019.J(2,2); 
Jz =  DE2019.J(3,3); 
 
nu_p_hat = 1/Jx * (L - q * r * Jz +  q * r * Jy ); 
nu_q_hat = 1/Jy *(M - r * p * Jx + r * p * Jz  );
nu_r_hat = 1/Jz * (N - p * q * Jy + p * q * Jx ); 

%------------- END CODE --------------
end

== matlab function Dyn_6DoF_v2_0_R2015B/AirborneSystem/FlightControlSystem/AttitudeAndRateLoop/RateLoop/Rate_Loop/InversionRotationalDynamics ==
  data: omega_OB_B input; M_des output; nu_NDI input; DE2019 parameter
% Copyright 2021 Delft University of Technology
%
% Licensed under the Apache License, Version 2.0 (the "License");
% you may not use this file except in compliance with the License.
% You may obtain a copy of the License at
%
%      http://www.apache.org/licenses/LICENSE-2.0
%
% Unless required by applicable law or agreed to in writing, software
% distributed under the License is distributed on an "AS IS" BASIS,
% WITHOUT WARRANTIES OR CONDITIONS OF ANY KIND, either express or implied.
% See the License for the specific language governing permissions and
% limitations under the License.

function M_des  = Rate_inv(omega_OB_B,nu_NDI,  DE2019)
%Rate_inv - Determine desired moments
%
% Inputs:
%    omega_OB_B - Commanded roll, pitch and yaw rates
%    nu_NDI     - Roll, pitch and yaw rate error incl. controller gains
%    DE2019     - Aircraft parameters
%
% Outputs:
%    M_des  - Expected roll rate error
%
% Other m-files required:   none
% Subfunctions:             none
% MAT-files required:       none
%
% Author: Sebastian Rapp, Ph.D., Revised by: Dylan Eijkelhof, M.Sc.
% Delft University of Technology
% email address: d.eijkelhof@tudelft.nl
% December 2019; Last revision: 19-March-2021

%------------- BEGIN CODE --------------

p = omega_OB_B(1); 
q = omega_OB_B(2); 
r = omega_OB_B(3); 

nu_p = nu_NDI(1); 
nu_q = nu_NDI(2); 
nu_r = nu_NDI(3); 
 
Jx = DE2019.J(1,1); 
Jy = DE2019.J(2,2); 
Jz = DE2019.J(3,3);

Lc = Jx * nu_p + q * r * Jz  - q * r * Jy; 
Mc = Jy * nu_q + r * p * Jx - r * p * Jz;
Nc = Jz * nu_r + p * q * Jy - p * q * Jx; 

M_des = [Lc; Mc; Nc];

%------------- END CODE --------------
end

== matlab function Dyn_6DoF_v2_0_R2015B/AirborneSystem/ForcesAndTorques/aerodynamic forces FSI/Rudder Aero/Rudder_aero ==
  data: input input double; out output double size=[6,1]; DE2019 parameter; ENVMT parameter
% Copyright 2021 Delft University of Technology
%
% Licensed under the Apache License, Version 2.0 (the "License");
% you may not use this file except in compliance with the License.
% You may obtain a copy of the License at
%
%      http://www.apache.org/licenses/LICENSE-2.0
%
% Unless required by applicable law or agreed to in writing, software
% distributed under the License is distributed on an "AS IS" BASIS,
% WITHOUT WARRANTIES OR CONDITIONS OF ANY KIND, either express or implied.
% See the License for the specific language governing permissions and
% limitations under the License.

function out = simpleAero(input, DE2019, ENVMT)
%simpleAero - Rudder simple aero calculation
%
% Inputs:
%    input  - airspeed, AoA, sideslip, CL and CD
%    DE2019 - Aircraft parameters
%    ENVMT  - Environment characteristics
%
% Outputs:
%    out    - 3D forces and moments generated by the rudder
%
%
% Author: Sebastian Rapp, Ph.D., Revised by: Dylan Eijkelhof, M.Sc.
% Delft University of Technology
% email address: d.eijkelhof@tudelft.nl
% December 2019; Last revision: 19-March-2021

%-------------	BEGIN CODE	--------------
    V = input(1);
    alpha = input(2);
    beta = input(3);

    q = 0.5*ENVMT.rhos*V^2;
   
    F_L_vs = 2*input(4)*q*DE2019.S_vs;
    F_D_vs = -2*input(5)*q*DE2019.S_vs;

    F_x_s = F_D_vs*cos(alpha)*cos(beta);
    F_y_s = -F_L_vs*cos(beta);
    F_z_s = 0;

    M_x_s = F_L_vs*(DE2019.b_vs*0.5);
    M_y_s = 0;
    M_z_s = F_L_vs*(DE2019.x_vs+DE2019.c_vs*0.25);

    out = [F_x_s, F_y_s, F_z_s, M_x_s, M_y_s, M_z_s]';
%-------------	END CODE	--------------  
end

== matlab function Dyn_6DoF_v2_0_R2015B/RequirementModelsAndLogging/Power_convergence/MATLAB Function ==
  settings: updateMethod=DISCRETE  sampleTime=simInit.Ts_power_conv_check
  data: flag output; m_new output; p_sum output; cnt output; flag input; m_old input; p_sum input; cnt input; u input; flightMode input; e_new output; e_old input; cnt_max_mat input; cnt_max_mat output; cycles_cnt input; cycles_cnt output
% Copyright 2021 Delft University of Technology
%
% Licensed under the Apache License, Version 2.0 (the "License");
% you may not use this file except in compliance with the License.
% You may obtain a copy of the License at
%
%      http://www.apache.org/licenses/LICENSE-2.0
%
% Unless required by applicable law or agreed to in writing, software
% distributed under the License is distributed on an "AS IS" BASIS,
% WITHOUT WARRANTIES OR CONDITIONS OF ANY KIND, either express or implied.
% See the License for the specific language governing permissions and
% limitations under the License.

function [flag, m_new, p_sum, cnt, e_new, cnt_max_mat,cycles_cnt] = fcn(flag, m_old, p_sum, cnt, u, flightMode, e_old,cnt_max_mat,cycles_cnt)
% function [flag, m_new, p_sum, cnt, e_new, cnt_max_mat,cycles_cnt] = fcn(flag, m_old, p_sum, cnt, u, flightMode, e_old,cnt_max_mat,cycles_cnt, cnt_extra)
%y = [u;old(1:end-1)];
% if cnt > nmax
%     new_mean = mean(y);
%     cnt = 0;
% end
p_sum = p_sum + u;
cnt = cnt + 1;

if flightMode == 5 && flag
    cnt_max_mat = cnt; 
    m_new = p_sum/cnt;
    cnt  = 0;
    cycles_cnt = cycles_cnt + 1;
    p_sum = 0;
    flag = 0;
    e_new = abs( m_new - m_old );
elseif flightMode == 6
%     if cnt_extra == 0 || cycles_cnt == 0
%         cycles_cnt = cycles_cnt + 1;
%     end
    flag = 1;
    m_new = m_old;
    e_new = e_old;
else
    flag = 0;
    m_new = m_old;
    e_new = e_old;
end

% m_new = m_old + (u-old(nmax))/nmax;
